simulink model "REFvsFI"  (R2023a)
settings: Solver=FixedStepAuto  StartTime=0.0  StopTime=T  RelTol=1e-3  EnableMultiTasking=on
values from neighbouring files (symbols this model uses):
  Ts = 1    [TestDataGen.m]
libraries: My_FI_Operations x114, simulink x2
(part 4 of 5)

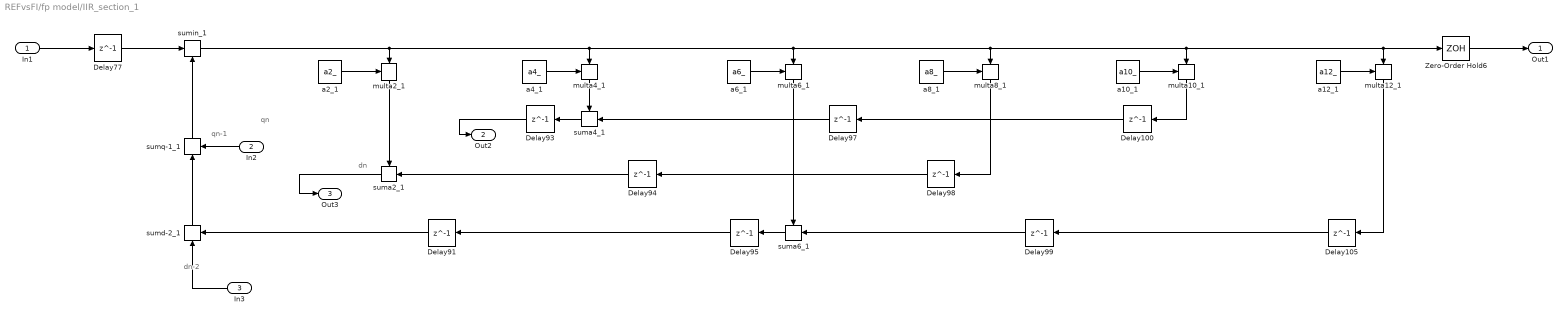
== system REFvsFI/fp model/IIR_section_1 ==
  note: dn
  note: dn-2
  note: qn
  note: qn-1
  In1 : Inport
  In2 : Inport  Port=2
  In3 : Inport  Port=3
  Delay{77,91,93..95,97..100,105} (10 alike) : Delay  DelayLength=1  SampleTime=3*Ts
  Zero-Order Hold6 : ZeroOrderHold  SampleTime=3*Ts
  a10_1 : My_FI_Operations/a10_  SystemSampleTime=-1  VariantActivationTime=update diagram  Latency=0  AutoFrameSizeCalculation=off
  a12_1 : My_FI_Operations/a12_  SystemSampleTime=-1  VariantActivationTime=update diagram  Latency=0  AutoFrameSizeCalculation=off
  a2_1 : My_FI_Operations/a2_  SystemSampleTime=-1  VariantActivationTime=update diagram  Latency=0  AutoFrameSizeCalculation=off
  a4_1 : My_FI_Operations/a4_  SystemSampleTime=-1  VariantActivationTime=update diagram  Latency=0  AutoFrameSizeCalculation=off
  a6_1 : My_FI_Operations/a6_  SystemSampleTime=-1  VariantActivationTime=update diagram  Latency=0  AutoFrameSizeCalculation=off
  a8_1 : My_FI_Operations/a8_  SystemSampleTime=-1  VariantActivationTime=update diagram  Latency=0  AutoFrameSizeCalculation=off
  multa10_1 : My_FI_Operations/multa10_  SystemSampleTime=-1  VariantActivationTime=update diagram  Latency=0  AutoFrameSizeCalculation=off
      settings: PortSchema="{\"entries\":[{\"content\":{\"sides\":[{\"content\":{\"connectorIds\":[\"In1\"]},\"type\":\"ConnectorPlacement.EquallySpacedRectSide\",\"uuid\":\"423828e0-6700-4575-ac06-a5fb7cb5569f\"},{\"content\":{\"connectorIds\":[],\"side\":\"RIGHT\"},\"type\":\"ConnectorPlacement.EquallySpacedRectSide\",\"uuid\":\"a42db842-eb55-44f2-8f04-0144bc45d908\"},{\"content\":{\"connectorIds\":[\"In2\"],\"side\":\"TOP\"},\"type\":\"ConnectorPlacement.EquallySpacedRectSide\",\"uuid\":\"eef5137d-31f0-46b4-a53b-5aa31464a7f9\"},{\"content\":{\"connectorIds\":[\"Out1\"],\"side\":\"BOTTOM\"},\"type\":\"ConnectorPlacement.EquallySpacedRectSide\",\"uuid\":\"0c804fa9-8d94-49f3-91d8-5fb511150c33\"}]},\"type\":\"ConnectorPlacement.EquallySpacedConnector\",\"uuid\":\"7dd7fe03-b221-4701-a7b2-6552f08320da\"}],\"packageUris\":[\"http://schema.mathworks.com/mf0/Connector/R2020b\"],\"version\":\"1.0\"}"
  multa12_1 : My_FI_Operations/multa12_  SystemSampleTime=-1  VariantActivationTime=update diagram  Latency=0  AutoFrameSizeCalculation=off
      settings: PortSchema="{\"entries\":[{\"content\":{\"sides\":[{\"content\":{\"connectorIds\":[\"In1\"]},\"type\":\"ConnectorPlacement.EquallySpacedRectSide\",\"uuid\":\"423828e0-6700-4575-ac06-a5fb7cb5569f\"},{\"content\":{\"connectorIds\":[],\"side\":\"RIGHT\"},\"type\":\"ConnectorPlacement.EquallySpacedRectSide\",\"uuid\":\"a42db842-eb55-44f2-8f04-0144bc45d908\"},{\"content\":{\"connectorIds\":[\"In2\"],\"side\":\"TOP\"},\"type\":\"ConnectorPlacement.EquallySpacedRectSide\",\"uuid\":\"eef5137d-31f0-46b4-a53b-5aa31464a7f9\"},{\"content\":{\"connectorIds\":[\"Out1\"],\"side\":\"BOTTOM\"},\"type\":\"ConnectorPlacement.EquallySpacedRectSide\",\"uuid\":\"8449918d-02c6-4967-8b4f-9e277713318d\"}]},\"type\":\"ConnectorPlacement.EquallySpacedConnector\",\"uuid\":\"7dd7fe03-b221-4701-a7b2-6552f08320da\"}],\"packageUris\":[\"http://schema.mathworks.com/mf0/Connector/R2020b\"],\"version\":\"1.0\"}"
  multa2_1 : My_FI_Operations/multa2_  SystemSampleTime=-1  VariantActivationTime=update diagram  Latency=0  AutoFrameSizeCalculation=off
      settings: PortSchema="{\"entries\":[{\"content\":{\"sides\":[{\"content\":{\"connectorIds\":[\"In1\"]},\"type\":\"ConnectorPlacement.EquallySpacedRectSide\",\"uuid\":\"423828e0-6700-4575-ac06-a5fb7cb5569f\"},{\"content\":{\"connectorIds\":[],\"side\":\"RIGHT\"},\"type\":\"ConnectorPlacement.EquallySpacedRectSide\",\"uuid\":\"a42db842-eb55-44f2-8f04-0144bc45d908\"},{\"content\":{\"connectorIds\":[\"In2\"],\"side\":\"TOP\"},\"type\":\"ConnectorPlacement.EquallySpacedRectSide\",\"uuid\":\"eef5137d-31f0-46b4-a53b-5aa31464a7f9\"},{\"content\":{\"connectorIds\":[\"Out1\"],\"side\":\"BOTTOM\"},\"type\":\"ConnectorPlacement.EquallySpacedRectSide\",\"uuid\":\"55d96b2a-2b7e-4fdf-a401-8e78f7d2a1aa\"}]},\"type\":\"ConnectorPlacement.EquallySpacedConnector\",\"uuid\":\"7dd7fe03-b221-4701-a7b2-6552f08320da\"}],\"packageUris\":[\"http://schema.mathworks.com/mf0/Connector/R2020b\"],\"version\":\"1.0\"}"
  multa4_1 : My_FI_Operations/multa4_  SystemSampleTime=-1  VariantActivationTime=update diagram  Latency=0  AutoFrameSizeCalculation=off
      settings: PortSchema="{\"entries\":[{\"content\":{\"sides\":[{\"content\":{\"connectorIds\":[\"In1\"]},\"type\":\"ConnectorPlacement.EquallySpacedRectSide\",\"uuid\":\"423828e0-6700-4575-ac06-a5fb7cb5569f\"},{\"content\":{\"connectorIds\":[],\"side\":\"RIGHT\"},\"type\":\"ConnectorPlacement.EquallySpacedRectSide\",\"uuid\":\"a42db842-eb55-44f2-8f04-0144bc45d908\"},{\"content\":{\"connectorIds\":[\"In2\"],\"side\":\"TOP\"},\"type\":\"ConnectorPlacement.EquallySpacedRectSide\",\"uuid\":\"eef5137d-31f0-46b4-a53b-5aa31464a7f9\"},{\"content\":{\"connectorIds\":[\"Out1\"],\"side\":\"BOTTOM\"},\"type\":\"ConnectorPlacement.EquallySpacedRectSide\",\"uuid\":\"24a9476e-4370-431a-bbc5-245c90c7a6e7\"}]},\"type\":\"ConnectorPlacement.EquallySpacedConnector\",\"uuid\":\"7dd7fe03-b221-4701-a7b2-6552f08320da\"}],\"packageUris\":[\"http://schema.mathworks.com/mf0/Connector/R2020b\"],\"version\":\"1.0\"}"
  multa6_1 : My_FI_Operations/multa6_  SystemSampleTime=-1  VariantActivationTime=update diagram  Latency=0  AutoFrameSizeCalculation=off
      settings: PortSchema="{\"entries\":[{\"content\":{\"sides\":[{\"content\":{\"connectorIds\":[\"In1\"]},\"type\":\"ConnectorPlacement.EquallySpacedRectSide\",\"uuid\":\"423828e0-6700-4575-ac06-a5fb7cb5569f\"},{\"content\":{\"connectorIds\":[],\"side\":\"RIGHT\"},\"type\":\"ConnectorPlacement.EquallySpacedRectSide\",\"uuid\":\"a42db842-eb55-44f2-8f04-0144bc45d908\"},{\"content\":{\"connectorIds\":[\"In2\"],\"side\":\"TOP\"},\"type\":\"ConnectorPlacement.EquallySpacedRectSide\",\"uuid\":\"eef5137d-31f0-46b4-a53b-5aa31464a7f9\"},{\"content\":{\"connectorIds\":[\"Out1\"],\"side\":\"BOTTOM\"},\"type\":\"ConnectorPlacement.EquallySpacedRectSide\",\"uuid\":\"47329aef-84bb-47a0-9b32-b12909a392a1\"}]},\"type\":\"ConnectorPlacement.EquallySpacedConnector\",\"uuid\":\"7dd7fe03-b221-4701-a7b2-6552f08320da\"}],\"packageUris\":[\"http://schema.mathworks.com/mf0/Connector/R2020b\"],\"version\":\"1.0\"}"
  multa8_1 : My_FI_Operations/multa8_  SystemSampleTime=-1  VariantActivationTime=update diagram  Latency=0  AutoFrameSizeCalculation=off
      settings: PortSchema="{\"entries\":[{\"content\":{\"sides\":[{\"content\":{\"connectorIds\":[\"In1\"]},\"type\":\"ConnectorPlacement.EquallySpacedRectSide\",\"uuid\":\"423828e0-6700-4575-ac06-a5fb7cb5569f\"},{\"content\":{\"connectorIds\":[],\"side\":\"RIGHT\"},\"type\":\"ConnectorPlacement.EquallySpacedRectSide\",\"uuid\":\"a42db842-eb55-44f2-8f04-0144bc45d908\"},{\"content\":{\"connectorIds\":[\"In2\"],\"side\":\"TOP\"},\"type\":\"ConnectorPlacement.EquallySpacedRectSide\",\"uuid\":\"eef5137d-31f0-46b4-a53b-5aa31464a7f9\"},{\"content\":{\"connectorIds\":[\"Out1\"],\"side\":\"BOTTOM\"},\"type\":\"ConnectorPlacement.EquallySpacedRectSide\",\"uuid\":\"5c073f60-f22f-4cd7-abc5-d0d5f88f0213\"}]},\"type\":\"ConnectorPlacement.EquallySpacedConnector\",\"uuid\":\"7dd7fe03-b221-4701-a7b2-6552f08320da\"}],\"packageUris\":[\"http://schema.mathworks.com/mf0/Connector/R2020b\"],\"version\":\"1.0\"}"
  suma2_1 : My_FI_Operations/suma2_  SystemSampleTime=-1  VariantActivationTime=update diagram  Latency=0  AutoFrameSizeCalculation=off
      settings: PortSchema="{\"entries\":[{\"content\":{\"sides\":[{\"content\":{\"connectorIds\":[\"Out1\"]},\"type\":\"ConnectorPlacement.EquallySpacedRectSide\",\"uuid\":\"423828e0-6700-4575-ac06-a5fb7cb5569f\"},{\"content\":{\"connectorIds\":[\"In2\"],\"side\":\"RIGHT\"},\"type\":\"ConnectorPlacement.EquallySpacedRectSide\",\"uuid\":\"a42db842-eb55-44f2-8f04-0144bc45d908\"},{\"content\":{\"connectorIds\":[\"In1\"],\"side\":\"TOP\"},\"type\":\"ConnectorPlacement.EquallySpacedRectSide\",\"uuid\":\"eef5137d-31f0-46b4-a53b-5aa31464a7f9\"}]},\"type\":\"ConnectorPlacement.EquallySpacedConnector\",\"uuid\":\"7dd7fe03-b221-4701-a7b2-6552f08320da\"}],\"packageUris\":[\"http://schema.mathworks.com/mf0/Connector/R2020b\"],\"version\":\"1.0\"}"
  suma4_1 : My_FI_Operations/suma4_  SystemSampleTime=-1  VariantActivationTime=update diagram  Latency=0  AutoFrameSizeCalculation=off
      settings: PortSchema="{\"entries\":[{\"content\":{\"sides\":[{\"content\":{\"connectorIds\":[\"Out1\"]},\"type\":\"ConnectorPlacement.EquallySpacedRectSide\",\"uuid\":\"423828e0-6700-4575-ac06-a5fb7cb5569f\"},{\"content\":{\"connectorIds\":[\"In2\"],\"side\":\"RIGHT\"},\"type\":\"ConnectorPlacement.EquallySpacedRectSide\",\"uuid\":\"a42db842-eb55-44f2-8f04-0144bc45d908\"},{\"content\":{\"connectorIds\":[\"In1\"],\"side\":\"TOP\"},\"type\":\"ConnectorPlacement.EquallySpacedRectSide\",\"uuid\":\"eef5137d-31f0-46b4-a53b-5aa31464a7f9\"}]},\"type\":\"ConnectorPlacement.EquallySpacedConnector\",\"uuid\":\"7dd7fe03-b221-4701-a7b2-6552f08320da\"}],\"packageUris\":[\"http://schema.mathworks.com/mf0/Connector/R2020b\"],\"version\":\"1.0\"}"
  suma6_1 : My_FI_Operations/suma6_  SystemSampleTime=-1  VariantActivationTime=update diagram  Latency=0  AutoFrameSizeCalculation=off
      settings: PortSchema="{\"entries\":[{\"content\":{\"sides\":[{\"content\":{\"connectorIds\":[\"Out1\"]},\"type\":\"ConnectorPlacement.EquallySpacedRectSide\",\"uuid\":\"423828e0-6700-4575-ac06-a5fb7cb5569f\"},{\"content\":{\"connectorIds\":[\"In2\"],\"side\":\"RIGHT\"},\"type\":\"ConnectorPlacement.EquallySpacedRectSide\",\"uuid\":\"a42db842-eb55-44f2-8f04-0144bc45d908\"},{\"content\":{\"connectorIds\":[\"In1\"],\"side\":\"TOP\"},\"type\":\"ConnectorPlacement.EquallySpacedRectSide\",\"uuid\":\"eef5137d-31f0-46b4-a53b-5aa31464a7f9\"}]},\"type\":\"ConnectorPlacement.EquallySpacedConnector\",\"uuid\":\"7dd7fe03-b221-4701-a7b2-6552f08320da\"}],\"packageUris\":[\"http://schema.mathworks.com/mf0/Connector/R2020b\"],\"version\":\"1.0\"}"
  sumd-2_1 : My_FI_Operations/sumd-2_  SystemSampleTime=-1  VariantActivationTime=update diagram  Latency=0  AutoFrameSizeCalculation=off
      settings: PortSchema="{\"entries\":[{\"content\":{\"sides\":[{\"content\":{\"connectorIds\":[]},\"type\":\"ConnectorPlacement.EquallySpacedRectSide\",\"uuid\":\"423828e0-6700-4575-ac06-a5fb7cb5569f\"},{\"content\":{\"connectorIds\":[\"In2\"],\"side\":\"RIGHT\"},\"type\":\"ConnectorPlacement.EquallySpacedRectSide\",\"uuid\":\"a42db842-eb55-44f2-8f04-0144bc45d908\"},{\"content\":{\"connectorIds\":[\"Out1\"],\"side\":\"TOP\"},\"type\":\"ConnectorPlacement.EquallySpacedRectSide\",\"uuid\":\"eef5137d-31f0-46b4-a53b-5aa31464a7f9\"},{\"content\":{\"connectorIds\":[\"In1\"],\"side\":\"BOTTOM\"},\"type\":\"ConnectorPlacement.EquallySpacedRectSide\",\"uuid\":\"0a29e77a-4bdf-45d0-8a25-1103c3446174\"}]},\"type\":\"ConnectorPlacement.EquallySpacedConnector\",\"uuid\":\"7dd7fe03-b221-4701-a7b2-6552f08320da\"}],\"packageUris\":[\"http://schema.mathworks.com/mf0/Connector/R2020b\"],\"version\":\"1.0\"}"
  sumin_1 : My_FI_Operations/sumin_  SystemSampleTime=-1  VariantActivationTime=update diagram  Latency=0  AutoFrameSizeCalculation=off
      settings: PortSchema="{\"entries\":[{\"content\":{\"sides\":[{\"content\":{\"connectorIds\":[\"In1\"]},\"type\":\"ConnectorPlacement.EquallySpacedRectSide\",\"uuid\":\"423828e0-6700-4575-ac06-a5fb7cb5569f\"},{\"content\":{\"connectorIds\":[\"Out1\"],\"side\":\"RIGHT\"},\"type\":\"ConnectorPlacement.EquallySpacedRectSide\",\"uuid\":\"a42db842-eb55-44f2-8f04-0144bc45d908\"},{\"content\":{\"connectorIds\":[],\"side\":\"TOP\"},\"type\":\"ConnectorPlacement.EquallySpacedRectSide\",\"uuid\":\"eef5137d-31f0-46b4-a53b-5aa31464a7f9\"},{\"content\":{\"connectorIds\":[\"In2\"],\"side\":\"BOTTOM\"},\"type\":\"ConnectorPlacement.EquallySpacedRectSide\",\"uuid\":\"f3760898-0e2b-4385-8757-2cc61988fa54\"}]},\"type\":\"ConnectorPlacement.EquallySpacedConnector\",\"uuid\":\"7dd7fe03-b221-4701-a7b2-6552f08320da\"}],\"packageUris\":[\"http://schema.mathworks.com/mf0/Connector/R2020b\"],\"version\":\"1.0\"}"
  sumq-1_1 : My_FI_Operations/sumq-1_  SystemSampleTime=-1  VariantActivationTime=update diagram  Latency=0  AutoFrameSizeCalculation=off
      settings: PortSchema="{\"entries\":[{\"content\":{\"sides\":[{\"content\":{\"connectorIds\":[]},\"type\":\"ConnectorPlacement.EquallySpacedRectSide\",\"uuid\":\"423828e0-6700-4575-ac06-a5fb7cb5569f\"},{\"content\":{\"connectorIds\":[\"In2\"],\"side\":\"RIGHT\"},\"type\":\"ConnectorPlacement.EquallySpacedRectSide\",\"uuid\":\"a42db842-eb55-44f2-8f04-0144bc45d908\"},{\"content\":{\"connectorIds\":[\"Out1\"],\"side\":\"TOP\"},\"type\":\"ConnectorPlacement.EquallySpacedRectSide\",\"uuid\":\"eef5137d-31f0-46b4-a53b-5aa31464a7f9\"},{\"content\":{\"connectorIds\":[\"In1\"],\"side\":\"BOTTOM\"},\"type\":\"ConnectorPlacement.EquallySpacedRectSide\",\"uuid\":\"2873f229-5340-47da-9b40-109923f96826\"}]},\"type\":\"ConnectorPlacement.EquallySpacedConnector\",\"uuid\":\"7dd7fe03-b221-4701-a7b2-6552f08320da\"}],\"packageUris\":[\"http://schema.mathworks.com/mf0/Connector/R2020b\"],\"version\":\"1.0\"}"
  Out1 : Outport
  Out2 : Outport  Port=2
  Out3 : Outport  Port=3
  wires:
  Delay77/1 -> sumin_1/1
  a12_1/1 -> multa12_1/1
  Delay98/1 -> Delay94/1
  Delay91/1 -> sumd-2_1/2
  sumin_1/1 -> multa2_1/2, multa4_1/2, multa6_1/2, multa8_1/2, multa10_1/2, multa12_1/2, Zero-Order Hold6/1
  Delay99/1 -> suma6_1/2
  Delay95/1 -> Delay91/1
  Delay94/1 -> suma2_1/2
  sumd-2_1/1 -> sumq-1_1/1
  a2_1/1 -> multa2_1/1
  multa4_1/1 -> suma4_1/1
  Delay100/1 -> Delay97/1
  Zero-Order Hold6/1 -> Out1/1
  multa6_1/1 -> suma6_1/1
  a10_1/1 -> multa10_1/1
  a4_1/1 -> multa4_1/1
  multa12_1/1 -> Delay105/1
  multa2_1/1 -> suma2_1/1
  Delay105/1 -> Delay99/1
  a8_1/1 -> multa8_1/1
  suma6_1/1 -> Delay95/1
  Delay97/1 -> suma4_1/2
  multa10_1/1 -> Delay100/1
  suma4_1/1 -> Delay93/1
  multa8_1/1 -> Delay98/1
  Delay93/1 -> Out2/1
  sumq-1_1/1 -> sumin_1/2
  a6_1/1 -> multa6_1/1
  In2/1 -> sumq-1_1/2
  In1/1 -> Delay77/1
  In3/1 -> sumd-2_1/1
  suma2_1/1 -> Out3/1

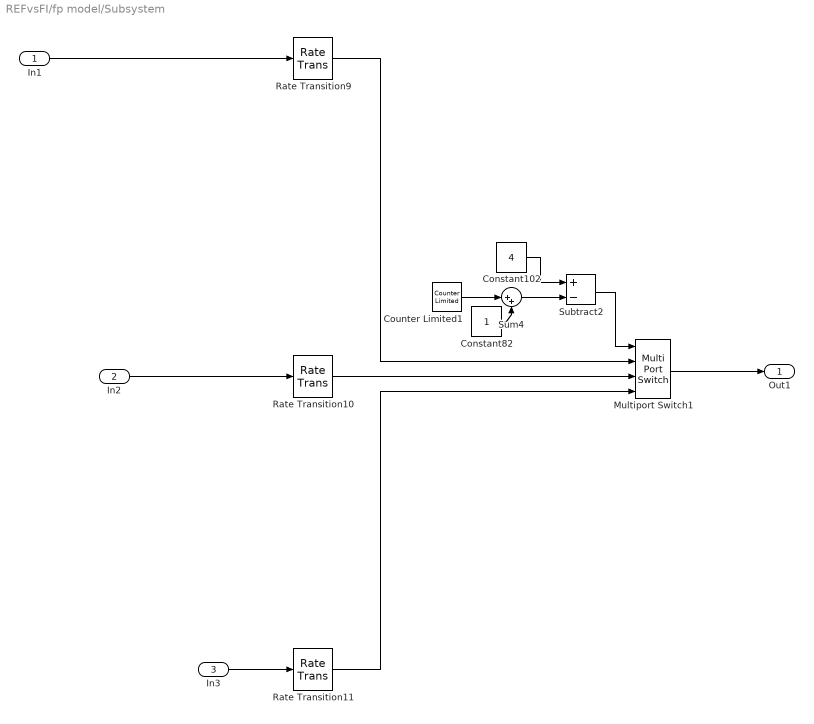
== system REFvsFI/fp model/Subsystem ==
  In1 : Inport
  In2 : Inport  Port=2
  In3 : Inport  Port=3
  Constant102 : Constant  Value=4  OutDataTypeStr=fixdt(0,3,0)
  Constant82 : Constant  OutDataTypeStr=fixdt(0,1,0)
  Counter Limited1 : simulink/Sources/Counter Limited  uplimit=2  tsamp=Ts
  Multiport Switch1 : MultiPortSwitch  OutDataTypeStr=fixdt(1,WL,FLout)  RndMeth=Nearest  SaturateOnIntegerOverflow=off  InputSameDT=off
  Rate Transition10 : RateTransition  OutPortSampleTime=Ts
  Rate Transition11 : RateTransition  OutPortSampleTime=Ts
  Rate Transition9 : RateTransition  OutPortSampleTime=Ts
  Subtract2 : Sum  Inputs=+-  OutDataTypeStr=fixdt(0,2,0)
  Sum4 : Sum  Inputs=|++  OutDataTypeStr=fixdt(0,2,0)
  Out1 : Outport
  wires:
  Rate Transition11/1 -> Multiport Switch1/4
  Constant82/1 -> Sum4/2
  Subtract2/1 -> Multiport Switch1/1
  Counter Limited1/1 -> Sum4/1
  Sum4/1 -> Subtract2/2
  Constant102/1 -> Subtract2/1
  Rate Transition9/1 -> Multiport Switch1/2
  Rate Transition10/1 -> Multiport Switch1/3
  In2/1 -> Rate Transition10/1
  In1/1 -> Rate Transition9/1
  Multiport Switch1/1 -> Out1/1
  In3/1 -> Rate Transition11/1

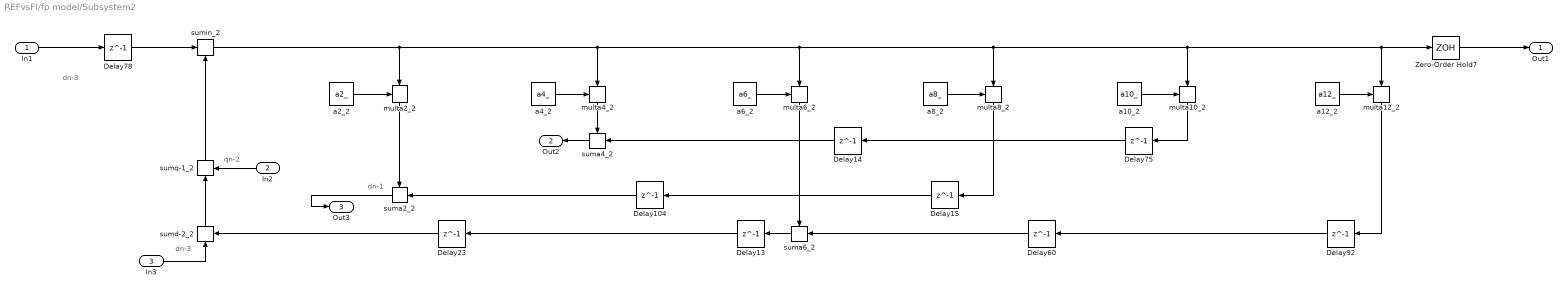
== system REFvsFI/fp model/Subsystem2 ==
  note: dn-1
  note: dn-3
  note: dn-3
  note: qn-2
  In1 : Inport
  In2 : Inport  Port=2
  In3 : Inport  Port=3
  Delay{13..15,23,60,75,78,92,104} (9 alike) : Delay  DelayLength=1  SampleTime=3*Ts
  Zero-Order Hold7 : ZeroOrderHold  SampleTime=3*Ts
  a10_2 : My_FI_Operations/a10_  SystemSampleTime=-1  VariantActivationTime=update diagram  Latency=0  AutoFrameSizeCalculation=off
  a12_2 : My_FI_Operations/a12_  SystemSampleTime=-1  VariantActivationTime=update diagram  Latency=0  AutoFrameSizeCalculation=off
  a2_2 : My_FI_Operations/a2_  SystemSampleTime=-1  VariantActivationTime=update diagram  Latency=0  AutoFrameSizeCalculation=off
  a4_2 : My_FI_Operations/a4_  SystemSampleTime=-1  VariantActivationTime=update diagram  Latency=0  AutoFrameSizeCalculation=off
  a6_2 : My_FI_Operations/a6_  SystemSampleTime=-1  VariantActivationTime=update diagram  Latency=0  AutoFrameSizeCalculation=off
  a8_2 : My_FI_Operations/a8_  SystemSampleTime=-1  VariantActivationTime=update diagram  Latency=0  AutoFrameSizeCalculation=off
  multa10_2 : My_FI_Operations/multa10_  SystemSampleTime=-1  VariantActivationTime=update diagram  Latency=0  AutoFrameSizeCalculation=off
      settings: PortSchema="{\"entries\":[{\"content\":{\"sides\":[{\"content\":{\"connectorIds\":[\"In1\"]},\"type\":\"ConnectorPlacement.EquallySpacedRectSide\",\"uuid\":\"423828e0-6700-4575-ac06-a5fb7cb5569f\"},{\"content\":{\"connectorIds\":[],\"side\":\"RIGHT\"},\"type\":\"ConnectorPlacement.EquallySpacedRectSide\",\"uuid\":\"a42db842-eb55-44f2-8f04-0144bc45d908\"},{\"content\":{\"connectorIds\":[\"In2\"],\"side\":\"TOP\"},\"type\":\"ConnectorPlacement.EquallySpacedRectSide\",\"uuid\":\"eef5137d-31f0-46b4-a53b-5aa31464a7f9\"},{\"content\":{\"connectorIds\":[\"Out1\"],\"side\":\"BOTTOM\"},\"type\":\"ConnectorPlacement.EquallySpacedRectSide\",\"uuid\":\"0c804fa9-8d94-49f3-91d8-5fb511150c33\"}]},\"type\":\"ConnectorPlacement.EquallySpacedConnector\",\"uuid\":\"7dd7fe03-b221-4701-a7b2-6552f08320da\"}],\"packageUris\":[\"http://schema.mathworks.com/mf0/Connector/R2020b\"],\"version\":\"1.0\"}"
  multa12_2 : My_FI_Operations/multa12_  SystemSampleTime=-1  VariantActivationTime=update diagram  Latency=0  AutoFrameSizeCalculation=off
      settings: PortSchema="{\"entries\":[{\"content\":{\"sides\":[{\"content\":{\"connectorIds\":[\"In1\"]},\"type\":\"ConnectorPlacement.EquallySpacedRectSide\",\"uuid\":\"423828e0-6700-4575-ac06-a5fb7cb5569f\"},{\"content\":{\"connectorIds\":[],\"side\":\"RIGHT\"},\"type\":\"ConnectorPlacement.EquallySpacedRectSide\",\"uuid\":\"a42db842-eb55-44f2-8f04-0144bc45d908\"},{\"content\":{\"connectorIds\":[\"In2\"],\"side\":\"TOP\"},\"type\":\"ConnectorPlacement.EquallySpacedRectSide\",\"uuid\":\"eef5137d-31f0-46b4-a53b-5aa31464a7f9\"},{\"content\":{\"connectorIds\":[\"Out1\"],\"side\":\"BOTTOM\"},\"type\":\"ConnectorPlacement.EquallySpacedRectSide\",\"uuid\":\"8449918d-02c6-4967-8b4f-9e277713318d\"}]},\"type\":\"ConnectorPlacement.EquallySpacedConnector\",\"uuid\":\"7dd7fe03-b221-4701-a7b2-6552f08320da\"}],\"packageUris\":[\"http://schema.mathworks.com/mf0/Connector/R2020b\"],\"version\":\"1.0\"}"
  multa2_2 : My_FI_Operations/multa2_  SystemSampleTime=-1  VariantActivationTime=update diagram  Latency=0  AutoFrameSizeCalculation=off
      settings: PortSchema="{\"entries\":[{\"content\":{\"sides\":[{\"content\":{\"connectorIds\":[\"In1\"]},\"type\":\"ConnectorPlacement.EquallySpacedRectSide\",\"uuid\":\"423828e0-6700-4575-ac06-a5fb7cb5569f\"},{\"content\":{\"connectorIds\":[],\"side\":\"RIGHT\"},\"type\":\"ConnectorPlacement.EquallySpacedRectSide\",\"uuid\":\"a42db842-eb55-44f2-8f04-0144bc45d908\"},{\"content\":{\"connectorIds\":[\"In2\"],\"side\":\"TOP\"},\"type\":\"ConnectorPlacement.EquallySpacedRectSide\",\"uuid\":\"eef5137d-31f0-46b4-a53b-5aa31464a7f9\"},{\"content\":{\"connectorIds\":[\"Out1\"],\"side\":\"BOTTOM\"},\"type\":\"ConnectorPlacement.EquallySpacedRectSide\",\"uuid\":\"55d96b2a-2b7e-4fdf-a401-8e78f7d2a1aa\"}]},\"type\":\"ConnectorPlacement.EquallySpacedConnector\",\"uuid\":\"7dd7fe03-b221-4701-a7b2-6552f08320da\"}],\"packageUris\":[\"http://schema.mathworks.com/mf0/Connector/R2020b\"],\"version\":\"1.0\"}"
  multa4_2 : My_FI_Operations/multa4_  SystemSampleTime=-1  VariantActivationTime=update diagram  Latency=0  AutoFrameSizeCalculation=off
      settings: PortSchema="{\"entries\":[{\"content\":{\"sides\":[{\"content\":{\"connectorIds\":[\"In1\"]},\"type\":\"ConnectorPlacement.EquallySpacedRectSide\",\"uuid\":\"423828e0-6700-4575-ac06-a5fb7cb5569f\"},{\"content\":{\"connectorIds\":[],\"side\":\"RIGHT\"},\"type\":\"ConnectorPlacement.EquallySpacedRectSide\",\"uuid\":\"a42db842-eb55-44f2-8f04-0144bc45d908\"},{\"content\":{\"connectorIds\":[\"In2\"],\"side\":\"TOP\"},\"type\":\"ConnectorPlacement.EquallySpacedRectSide\",\"uuid\":\"eef5137d-31f0-46b4-a53b-5aa31464a7f9\"},{\"content\":{\"connectorIds\":[\"Out1\"],\"side\":\"BOTTOM\"},\"type\":\"ConnectorPlacement.EquallySpacedRectSide\",\"uuid\":\"24a9476e-4370-431a-bbc5-245c90c7a6e7\"}]},\"type\":\"ConnectorPlacement.EquallySpacedConnector\",\"uuid\":\"7dd7fe03-b221-4701-a7b2-6552f08320da\"}],\"packageUris\":[\"http://schema.mathworks.com/mf0/Connector/R2020b\"],\"version\":\"1.0\"}"
  multa6_2 : My_FI_Operations/multa6_  SystemSampleTime=-1  VariantActivationTime=update diagram  Latency=0  AutoFrameSizeCalculation=off
      settings: PortSchema="{\"entries\":[{\"content\":{\"sides\":[{\"content\":{\"connectorIds\":[\"In1\"]},\"type\":\"ConnectorPlacement.EquallySpacedRectSide\",\"uuid\":\"423828e0-6700-4575-ac06-a5fb7cb5569f\"},{\"content\":{\"connectorIds\":[],\"side\":\"RIGHT\"},\"type\":\"ConnectorPlacement.EquallySpacedRectSide\",\"uuid\":\"a42db842-eb55-44f2-8f04-0144bc45d908\"},{\"content\":{\"connectorIds\":[\"In2\"],\"side\":\"TOP\"},\"type\":\"ConnectorPlacement.EquallySpacedRectSide\",\"uuid\":\"eef5137d-31f0-46b4-a53b-5aa31464a7f9\"},{\"content\":{\"connectorIds\":[\"Out1\"],\"side\":\"BOTTOM\"},\"type\":\"ConnectorPlacement.EquallySpacedRectSide\",\"uuid\":\"47329aef-84bb-47a0-9b32-b12909a392a1\"}]},\"type\":\"ConnectorPlacement.EquallySpacedConnector\",\"uuid\":\"7dd7fe03-b221-4701-a7b2-6552f08320da\"}],\"packageUris\":[\"http://schema.mathworks.com/mf0/Connector/R2020b\"],\"version\":\"1.0\"}"
  multa8_2 : My_FI_Operations/multa8_  SystemSampleTime=-1  VariantActivationTime=update diagram  Latency=0  AutoFrameSizeCalculation=off
      settings: PortSchema="{\"entries\":[{\"content\":{\"sides\":[{\"content\":{\"connectorIds\":[\"In1\"]},\"type\":\"ConnectorPlacement.EquallySpacedRectSide\",\"uuid\":\"423828e0-6700-4575-ac06-a5fb7cb5569f\"},{\"content\":{\"connectorIds\":[],\"side\":\"RIGHT\"},\"type\":\"ConnectorPlacement.EquallySpacedRectSide\",\"uuid\":\"a42db842-eb55-44f2-8f04-0144bc45d908\"},{\"content\":{\"connectorIds\":[\"In2\"],\"side\":\"TOP\"},\"type\":\"ConnectorPlacement.EquallySpacedRectSide\",\"uuid\":\"eef5137d-31f0-46b4-a53b-5aa31464a7f9\"},{\"content\":{\"connectorIds\":[\"Out1\"],\"side\":\"BOTTOM\"},\"type\":\"ConnectorPlacement.EquallySpacedRectSide\",\"uuid\":\"5c073f60-f22f-4cd7-abc5-d0d5f88f0213\"}]},\"type\":\"ConnectorPlacement.EquallySpacedConnector\",\"uuid\":\"7dd7fe03-b221-4701-a7b2-6552f08320da\"}],\"packageUris\":[\"http://schema.mathworks.com/mf0/Connector/R2020b\"],\"version\":\"1.0\"}"
  suma2_2 : My_FI_Operations/suma2_  SystemSampleTime=-1  VariantActivationTime=update diagram  Latency=0  AutoFrameSizeCalculation=off
      settings: PortSchema="{\"entries\":[{\"content\":{\"sides\":[{\"content\":{\"connectorIds\":[\"Out1\"]},\"type\":\"ConnectorPlacement.EquallySpacedRectSide\",\"uuid\":\"423828e0-6700-4575-ac06-a5fb7cb5569f\"},{\"content\":{\"connectorIds\":[\"In2\"],\"side\":\"RIGHT\"},\"type\":\"ConnectorPlacement.EquallySpacedRectSide\",\"uuid\":\"a42db842-eb55-44f2-8f04-0144bc45d908\"},{\"content\":{\"connectorIds\":[\"In1\"],\"side\":\"TOP\"},\"type\":\"ConnectorPlacement.EquallySpacedRectSide\",\"uuid\":\"eef5137d-31f0-46b4-a53b-5aa31464a7f9\"}]},\"type\":\"ConnectorPlacement.EquallySpacedConnector\",\"uuid\":\"7dd7fe03-b221-4701-a7b2-6552f08320da\"}],\"packageUris\":[\"http://schema.mathworks.com/mf0/Connector/R2020b\"],\"version\":\"1.0\"}"
  suma4_2 : My_FI_Operations/suma4_  SystemSampleTime=-1  VariantActivationTime=update diagram  Latency=0  AutoFrameSizeCalculation=off
      settings: PortSchema="{\"entries\":[{\"content\":{\"sides\":[{\"content\":{\"connectorIds\":[\"Out1\"]},\"type\":\"ConnectorPlacement.EquallySpacedRectSide\",\"uuid\":\"423828e0-6700-4575-ac06-a5fb7cb5569f\"},{\"content\":{\"connectorIds\":[\"In2\"],\"side\":\"RIGHT\"},\"type\":\"ConnectorPlacement.EquallySpacedRectSide\",\"uuid\":\"a42db842-eb55-44f2-8f04-0144bc45d908\"},{\"content\":{\"connectorIds\":[\"In1\"],\"side\":\"TOP\"},\"type\":\"ConnectorPlacement.EquallySpacedRectSide\",\"uuid\":\"eef5137d-31f0-46b4-a53b-5aa31464a7f9\"}]},\"type\":\"ConnectorPlacement.EquallySpacedConnector\",\"uuid\":\"7dd7fe03-b221-4701-a7b2-6552f08320da\"}],\"packageUris\":[\"http://schema.mathworks.com/mf0/Connector/R2020b\"],\"version\":\"1.0\"}"
  suma6_2 : My_FI_Operations/suma6_  SystemSampleTime=-1  VariantActivationTime=update diagram  Latency=0  AutoFrameSizeCalculation=off
      settings: PortSchema="{\"entries\":[{\"content\":{\"sides\":[{\"content\":{\"connectorIds\":[\"Out1\"]},\"type\":\"ConnectorPlacement.EquallySpacedRectSide\",\"uuid\":\"423828e0-6700-4575-ac06-a5fb7cb5569f\"},{\"content\":{\"connectorIds\":[\"In2\"],\"side\":\"RIGHT\"},\"type\":\"ConnectorPlacement.EquallySpacedRectSide\",\"uuid\":\"a42db842-eb55-44f2-8f04-0144bc45d908\"},{\"content\":{\"connectorIds\":[\"In1\"],\"side\":\"TOP\"},\"type\":\"ConnectorPlacement.EquallySpacedRectSide\",\"uuid\":\"eef5137d-31f0-46b4-a53b-5aa31464a7f9\"}]},\"type\":\"ConnectorPlacement.EquallySpacedConnector\",\"uuid\":\"7dd7fe03-b221-4701-a7b2-6552f08320da\"}],\"packageUris\":[\"http://schema.mathworks.com/mf0/Connector/R2020b\"],\"version\":\"1.0\"}"
  sumd-2_2 : My_FI_Operations/sumd-2_  SystemSampleTime=-1  VariantActivationTime=update diagram  Latency=0  AutoFrameSizeCalculation=off
      settings: PortSchema="{\"entries\":[{\"content\":{\"sides\":[{\"content\":{\"connectorIds\":[]},\"type\":\"ConnectorPlacement.EquallySpacedRectSide\",\"uuid\":\"423828e0-6700-4575-ac06-a5fb7cb5569f\"},{\"content\":{\"connectorIds\":[\"In2\"],\"side\":\"RIGHT\"},\"type\":\"ConnectorPlacement.EquallySpacedRectSide\",\"uuid\":\"a42db842-eb55-44f2-8f04-0144bc45d908\"},{\"content\":{\"connectorIds\":[\"Out1\"],\"side\":\"TOP\"},\"type\":\"ConnectorPlacement.EquallySpacedRectSide\",\"uuid\":\"eef5137d-31f0-46b4-a53b-5aa31464a7f9\"},{\"content\":{\"connectorIds\":[\"In1\"],\"side\":\"BOTTOM\"},\"type\":\"ConnectorPlacement.EquallySpacedRectSide\",\"uuid\":\"0a29e77a-4bdf-45d0-8a25-1103c3446174\"}]},\"type\":\"ConnectorPlacement.EquallySpacedConnector\",\"uuid\":\"7dd7fe03-b221-4701-a7b2-6552f08320da\"}],\"packageUris\":[\"http://schema.mathworks.com/mf0/Connector/R2020b\"],\"version\":\"1.0\"}"
  sumin_2 : My_FI_Operations/sumin_  SystemSampleTime=-1  VariantActivationTime=update diagram  Latency=0  AutoFrameSizeCalculation=off
      settings: PortSchema="{\"entries\":[{\"content\":{\"sides\":[{\"content\":{\"connectorIds\":[\"In1\"]},\"type\":\"ConnectorPlacement.EquallySpacedRectSide\",\"uuid\":\"423828e0-6700-4575-ac06-a5fb7cb5569f\"},{\"content\":{\"connectorIds\":[\"Out1\"],\"side\":\"RIGHT\"},\"type\":\"ConnectorPlacement.EquallySpacedRectSide\",\"uuid\":\"a42db842-eb55-44f2-8f04-0144bc45d908\"},{\"content\":{\"connectorIds\":[],\"side\":\"TOP\"},\"type\":\"ConnectorPlacement.EquallySpacedRectSide\",\"uuid\":\"eef5137d-31f0-46b4-a53b-5aa31464a7f9\"},{\"content\":{\"connectorIds\":[\"In2\"],\"side\":\"BOTTOM\"},\"type\":\"ConnectorPlacement.EquallySpacedRectSide\",\"uuid\":\"f3760898-0e2b-4385-8757-2cc61988fa54\"}]},\"type\":\"ConnectorPlacement.EquallySpacedConnector\",\"uuid\":\"7dd7fe03-b221-4701-a7b2-6552f08320da\"}],\"packageUris\":[\"http://schema.mathworks.com/mf0/Connector/R2020b\"],\"version\":\"1.0\"}"
  sumq-1_2 : My_FI_Operations/sumq-1_  SystemSampleTime=-1  VariantActivationTime=update diagram  Latency=0  AutoFrameSizeCalculation=off
      settings: PortSchema="{\"entries\":[{\"content\":{\"sides\":[{\"content\":{\"connectorIds\":[]},\"type\":\"ConnectorPlacement.EquallySpacedRectSide\",\"uuid\":\"423828e0-6700-4575-ac06-a5fb7cb5569f\"},{\"content\":{\"connectorIds\":[\"In2\"],\"side\":\"RIGHT\"},\"type\":\"ConnectorPlacement.EquallySpacedRectSide\",\"uuid\":\"a42db842-eb55-44f2-8f04-0144bc45d908\"},{\"content\":{\"connectorIds\":[\"Out1\"],\"side\":\"TOP\"},\"type\":\"ConnectorPlacement.EquallySpacedRectSide\",\"uuid\":\"eef5137d-31f0-46b4-a53b-5aa31464a7f9\"},{\"content\":{\"connectorIds\":[\"In1\"],\"side\":\"BOTTOM\"},\"type\":\"ConnectorPlacement.EquallySpacedRectSide\",\"uuid\":\"2873f229-5340-47da-9b40-109923f96826\"}]},\"type\":\"ConnectorPlacement.EquallySpacedConnector\",\"uuid\":\"7dd7fe03-b221-4701-a7b2-6552f08320da\"}],\"packageUris\":[\"http://schema.mathworks.com/mf0/Connector/R2020b\"],\"version\":\"1.0\"}"
  Out1 : Outport
  Out2 : Outport  Port=2
  Out3 : Outport  Port=3
  wires:
  sumin_2/1 -> multa2_2/2, multa12_2/2, Zero-Order Hold7/1, multa10_2/2, multa8_2/2, multa6_2/2, multa4_2/2
  In2/1 -> sumq-1_2/2
  a12_2/1 -> multa12_2/1
  Delay78/1 -> sumin_2/1
  sumd-2_2/1 -> sumq-1_2/1
  suma6_2/1 -> Delay13/1
  Zero-Order Hold7/1 -> Out1/1
  sumq-1_2/1 -> sumin_2/2
  Delay15/1 -> Delay104/1
  Delay13/1 -> Delay23/1
  a10_2/1 -> multa10_2/1
  suma4_2/1 -> Out2/1
  In3/1 -> sumd-2_2/1
  multa10_2/1 -> Delay75/1
  multa8_2/1 -> Delay15/1
  multa4_2/1 -> suma4_2/1
  multa2_2/1 -> suma2_2/1
  Delay14/1 -> suma4_2/2
  a2_2/1 -> multa2_2/1
  Delay60/1 -> suma6_2/2
  a8_2/1 -> multa8_2/1
  multa6_2/1 -> suma6_2/1
  Delay75/1 -> Delay14/1
  multa12_2/1 -> Delay92/1
  a4_2/1 -> multa4_2/1
  a6_2/1 -> multa6_2/1
  Delay23/1 -> sumd-2_2/2
  Delay104/1 -> suma2_2/2
  In1/1 -> Delay78/1
  Delay92/1 -> Delay60/1
  suma2_2/1 -> Out3/1

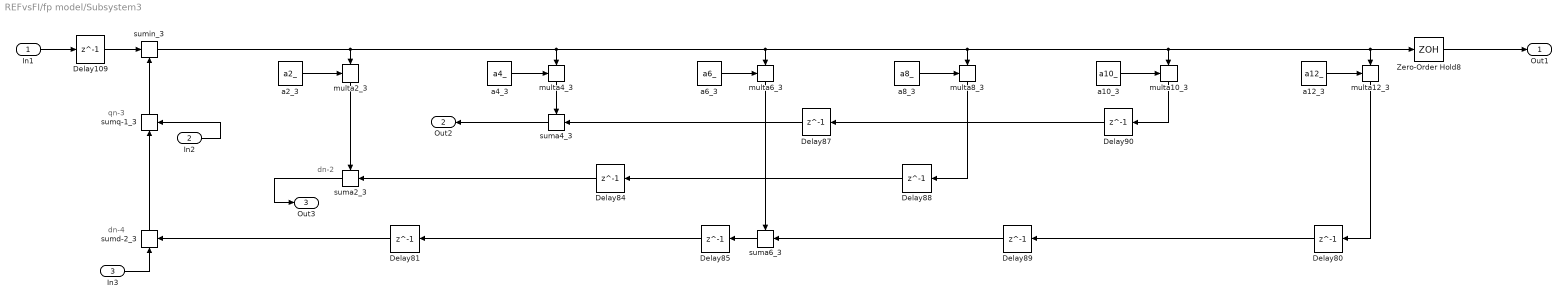
== system REFvsFI/fp model/Subsystem3 ==
  note: dn-2
  note: dn-4
  note: qn-3
  In1 : Inport
  In2 : Inport  Port=2
  In3 : Inport  Port=3
  Delay{80..81,84..85,87..90,109} (9 alike) : Delay  DelayLength=1  SampleTime=3*Ts
  Zero-Order Hold8 : ZeroOrderHold  SampleTime=3*Ts
  a10_3 : My_FI_Operations/a10_  SystemSampleTime=-1  VariantActivationTime=update diagram  Latency=0  AutoFrameSizeCalculation=off
  a12_3 : My_FI_Operations/a12_  SystemSampleTime=-1  VariantActivationTime=update diagram  Latency=0  AutoFrameSizeCalculation=off
  a2_3 : My_FI_Operations/a2_  SystemSampleTime=-1  VariantActivationTime=update diagram  Latency=0  AutoFrameSizeCalculation=off
  a4_3 : My_FI_Operations/a4_  SystemSampleTime=-1  VariantActivationTime=update diagram  Latency=0  AutoFrameSizeCalculation=off
  a6_3 : My_FI_Operations/a6_  SystemSampleTime=-1  VariantActivationTime=update diagram  Latency=0  AutoFrameSizeCalculation=off
  a8_3 : My_FI_Operations/a8_  SystemSampleTime=-1  VariantActivationTime=update diagram  Latency=0  AutoFrameSizeCalculation=off
  multa10_3 : My_FI_Operations/multa10_  SystemSampleTime=-1  VariantActivationTime=update diagram  Latency=0  AutoFrameSizeCalculation=off
      settings: PortSchema="{\"entries\":[{\"content\":{\"sides\":[{\"content\":{\"connectorIds\":[\"In1\"]},\"type\":\"ConnectorPlacement.EquallySpacedRectSide\",\"uuid\":\"423828e0-6700-4575-ac06-a5fb7cb5569f\"},{\"content\":{\"connectorIds\":[],\"side\":\"RIGHT\"},\"type\":\"ConnectorPlacement.EquallySpacedRectSide\",\"uuid\":\"a42db842-eb55-44f2-8f04-0144bc45d908\"},{\"content\":{\"connectorIds\":[\"In2\"],\"side\":\"TOP\"},\"type\":\"ConnectorPlacement.EquallySpacedRectSide\",\"uuid\":\"eef5137d-31f0-46b4-a53b-5aa31464a7f9\"},{\"content\":{\"connectorIds\":[\"Out1\"],\"side\":\"BOTTOM\"},\"type\":\"ConnectorPlacement.EquallySpacedRectSide\",\"uuid\":\"0c804fa9-8d94-49f3-91d8-5fb511150c33\"}]},\"type\":\"ConnectorPlacement.EquallySpacedConnector\",\"uuid\":\"7dd7fe03-b221-4701-a7b2-6552f08320da\"}],\"packageUris\":[\"http://schema.mathworks.com/mf0/Connector/R2020b\"],\"version\":\"1.0\"}"
  multa12_3 : My_FI_Operations/multa12_  SystemSampleTime=-1  VariantActivationTime=update diagram  Latency=0  AutoFrameSizeCalculation=off
      settings: PortSchema="{\"entries\":[{\"content\":{\"sides\":[{\"content\":{\"connectorIds\":[\"In1\"]},\"type\":\"ConnectorPlacement.EquallySpacedRectSide\",\"uuid\":\"423828e0-6700-4575-ac06-a5fb7cb5569f\"},{\"content\":{\"connectorIds\":[],\"side\":\"RIGHT\"},\"type\":\"ConnectorPlacement.EquallySpacedRectSide\",\"uuid\":\"a42db842-eb55-44f2-8f04-0144bc45d908\"},{\"content\":{\"connectorIds\":[\"In2\"],\"side\":\"TOP\"},\"type\":\"ConnectorPlacement.EquallySpacedRectSide\",\"uuid\":\"eef5137d-31f0-46b4-a53b-5aa31464a7f9\"},{\"content\":{\"connectorIds\":[\"Out1\"],\"side\":\"BOTTOM\"},\"type\":\"ConnectorPlacement.EquallySpacedRectSide\",\"uuid\":\"8449918d-02c6-4967-8b4f-9e277713318d\"}]},\"type\":\"ConnectorPlacement.EquallySpacedConnector\",\"uuid\":\"7dd7fe03-b221-4701-a7b2-6552f08320da\"}],\"packageUris\":[\"http://schema.mathworks.com/mf0/Connector/R2020b\"],\"version\":\"1.0\"}"
  multa2_3 : My_FI_Operations/multa2_  SystemSampleTime=-1  VariantActivationTime=update diagram  Latency=0  AutoFrameSizeCalculation=off
      settings: PortSchema="{\"entries\":[{\"content\":{\"sides\":[{\"content\":{\"connectorIds\":[\"In1\"]},\"type\":\"ConnectorPlacement.EquallySpacedRectSide\",\"uuid\":\"423828e0-6700-4575-ac06-a5fb7cb5569f\"},{\"content\":{\"connectorIds\":[],\"side\":\"RIGHT\"},\"type\":\"ConnectorPlacement.EquallySpacedRectSide\",\"uuid\":\"a42db842-eb55-44f2-8f04-0144bc45d908\"},{\"content\":{\"connectorIds\":[\"In2\"],\"side\":\"TOP\"},\"type\":\"ConnectorPlacement.EquallySpacedRectSide\",\"uuid\":\"eef5137d-31f0-46b4-a53b-5aa31464a7f9\"},{\"content\":{\"connectorIds\":[\"Out1\"],\"side\":\"BOTTOM\"},\"type\":\"ConnectorPlacement.EquallySpacedRectSide\",\"uuid\":\"55d96b2a-2b7e-4fdf-a401-8e78f7d2a1aa\"}]},\"type\":\"ConnectorPlacement.EquallySpacedConnector\",\"uuid\":\"7dd7fe03-b221-4701-a7b2-6552f08320da\"}],\"packageUris\":[\"http://schema.mathworks.com/mf0/Connector/R2020b\"],\"version\":\"1.0\"}"
  multa4_3 : My_FI_Operations/multa4_  SystemSampleTime=-1  VariantActivationTime=update diagram  Latency=0  AutoFrameSizeCalculation=off
      settings: PortSchema="{\"entries\":[{\"content\":{\"sides\":[{\"content\":{\"connectorIds\":[\"In1\"]},\"type\":\"ConnectorPlacement.EquallySpacedRectSide\",\"uuid\":\"423828e0-6700-4575-ac06-a5fb7cb5569f\"},{\"content\":{\"connectorIds\":[],\"side\":\"RIGHT\"},\"type\":\"ConnectorPlacement.EquallySpacedRectSide\",\"uuid\":\"a42db842-eb55-44f2-8f04-0144bc45d908\"},{\"content\":{\"connectorIds\":[\"In2\"],\"side\":\"TOP\"},\"type\":\"ConnectorPlacement.EquallySpacedRectSide\",\"uuid\":\"eef5137d-31f0-46b4-a53b-5aa31464a7f9\"},{\"content\":{\"connectorIds\":[\"Out1\"],\"side\":\"BOTTOM\"},\"type\":\"ConnectorPlacement.EquallySpacedRectSide\",\"uuid\":\"24a9476e-4370-431a-bbc5-245c90c7a6e7\"}]},\"type\":\"ConnectorPlacement.EquallySpacedConnector\",\"uuid\":\"7dd7fe03-b221-4701-a7b2-6552f08320da\"}],\"packageUris\":[\"http://schema.mathworks.com/mf0/Connector/R2020b\"],\"version\":\"1.0\"}"
  multa6_3 : My_FI_Operations/multa6_  SystemSampleTime=-1  VariantActivationTime=update diagram  Latency=0  AutoFrameSizeCalculation=off
      settings: PortSchema="{\"entries\":[{\"content\":{\"sides\":[{\"content\":{\"connectorIds\":[\"In1\"]},\"type\":\"ConnectorPlacement.EquallySpacedRectSide\",\"uuid\":\"423828e0-6700-4575-ac06-a5fb7cb5569f\"},{\"content\":{\"connectorIds\":[],\"side\":\"RIGHT\"},\"type\":\"ConnectorPlacement.EquallySpacedRectSide\",\"uuid\":\"a42db842-eb55-44f2-8f04-0144bc45d908\"},{\"content\":{\"connectorIds\":[\"In2\"],\"side\":\"TOP\"},\"type\":\"ConnectorPlacement.EquallySpacedRectSide\",\"uuid\":\"eef5137d-31f0-46b4-a53b-5aa31464a7f9\"},{\"content\":{\"connectorIds\":[\"Out1\"],\"side\":\"BOTTOM\"},\"type\":\"ConnectorPlacement.EquallySpacedRectSide\",\"uuid\":\"47329aef-84bb-47a0-9b32-b12909a392a1\"}]},\"type\":\"ConnectorPlacement.EquallySpacedConnector\",\"uuid\":\"7dd7fe03-b221-4701-a7b2-6552f08320da\"}],\"packageUris\":[\"http://schema.mathworks.com/mf0/Connector/R2020b\"],\"version\":\"1.0\"}"
  multa8_3 : My_FI_Operations/multa8_  SystemSampleTime=-1  VariantActivationTime=update diagram  Latency=0  AutoFrameSizeCalculation=off
      settings: PortSchema="{\"entries\":[{\"content\":{\"sides\":[{\"content\":{\"connectorIds\":[\"In1\"]},\"type\":\"ConnectorPlacement.EquallySpacedRectSide\",\"uuid\":\"423828e0-6700-4575-ac06-a5fb7cb5569f\"},{\"content\":{\"connectorIds\":[],\"side\":\"RIGHT\"},\"type\":\"ConnectorPlacement.EquallySpacedRectSide\",\"uuid\":\"a42db842-eb55-44f2-8f04-0144bc45d908\"},{\"content\":{\"connectorIds\":[\"In2\"],\"side\":\"TOP\"},\"type\":\"ConnectorPlacement.EquallySpacedRectSide\",\"uuid\":\"eef5137d-31f0-46b4-a53b-5aa31464a7f9\"},{\"content\":{\"connectorIds\":[\"Out1\"],\"side\":\"BOTTOM\"},\"type\":\"ConnectorPlacement.EquallySpacedRectSide\",\"uuid\":\"5c073f60-f22f-4cd7-abc5-d0d5f88f0213\"}]},\"type\":\"ConnectorPlacement.EquallySpacedConnector\",\"uuid\":\"7dd7fe03-b221-4701-a7b2-6552f08320da\"}],\"packageUris\":[\"http://schema.mathworks.com/mf0/Connector/R2020b\"],\"version\":\"1.0\"}"
  suma2_3 : My_FI_Operations/suma2_  SystemSampleTime=-1  VariantActivationTime=update diagram  Latency=0  AutoFrameSizeCalculation=off
      settings: PortSchema="{\"entries\":[{\"content\":{\"sides\":[{\"content\":{\"connectorIds\":[\"Out1\"]},\"type\":\"ConnectorPlacement.EquallySpacedRectSide\",\"uuid\":\"423828e0-6700-4575-ac06-a5fb7cb5569f\"},{\"content\":{\"connectorIds\":[\"In2\"],\"side\":\"RIGHT\"},\"type\":\"ConnectorPlacement.EquallySpacedRectSide\",\"uuid\":\"a42db842-eb55-44f2-8f04-0144bc45d908\"},{\"content\":{\"connectorIds\":[\"In1\"],\"side\":\"TOP\"},\"type\":\"ConnectorPlacement.EquallySpacedRectSide\",\"uuid\":\"eef5137d-31f0-46b4-a53b-5aa31464a7f9\"}]},\"type\":\"ConnectorPlacement.EquallySpacedConnector\",\"uuid\":\"7dd7fe03-b221-4701-a7b2-6552f08320da\"}],\"packageUris\":[\"http://schema.mathworks.com/mf0/Connector/R2020b\"],\"version\":\"1.0\"}"
  suma4_3 : My_FI_Operations/suma4_  SystemSampleTime=-1  VariantActivationTime=update diagram  Latency=0  AutoFrameSizeCalculation=off
      settings: PortSchema="{\"entries\":[{\"content\":{\"sides\":[{\"content\":{\"connectorIds\":[\"Out1\"]},\"type\":\"ConnectorPlacement.EquallySpacedRectSide\",\"uuid\":\"423828e0-6700-4575-ac06-a5fb7cb5569f\"},{\"content\":{\"connectorIds\":[\"In2\"],\"side\":\"RIGHT\"},\"type\":\"ConnectorPlacement.EquallySpacedRectSide\",\"uuid\":\"a42db842-eb55-44f2-8f04-0144bc45d908\"},{\"content\":{\"connectorIds\":[\"In1\"],\"side\":\"TOP\"},\"type\":\"ConnectorPlacement.EquallySpacedRectSide\",\"uuid\":\"eef5137d-31f0-46b4-a53b-5aa31464a7f9\"}]},\"type\":\"ConnectorPlacement.EquallySpacedConnector\",\"uuid\":\"7dd7fe03-b221-4701-a7b2-6552f08320da\"}],\"packageUris\":[\"http://schema.mathworks.com/mf0/Connector/R2020b\"],\"version\":\"1.0\"}"
  suma6_3 : My_FI_Operations/suma6_  SystemSampleTime=-1  VariantActivationTime=update diagram  Latency=0  AutoFrameSizeCalculation=off
      settings: PortSchema="{\"entries\":[{\"content\":{\"sides\":[{\"content\":{\"connectorIds\":[\"Out1\"]},\"type\":\"ConnectorPlacement.EquallySpacedRectSide\",\"uuid\":\"423828e0-6700-4575-ac06-a5fb7cb5569f\"},{\"content\":{\"connectorIds\":[\"In2\"],\"side\":\"RIGHT\"},\"type\":\"ConnectorPlacement.EquallySpacedRectSide\",\"uuid\":\"a42db842-eb55-44f2-8f04-0144bc45d908\"},{\"content\":{\"connectorIds\":[\"In1\"],\"side\":\"TOP\"},\"type\":\"ConnectorPlacement.EquallySpacedRectSide\",\"uuid\":\"eef5137d-31f0-46b4-a53b-5aa31464a7f9\"}]},\"type\":\"ConnectorPlacement.EquallySpacedConnector\",\"uuid\":\"7dd7fe03-b221-4701-a7b2-6552f08320da\"}],\"packageUris\":[\"http://schema.mathworks.com/mf0/Connector/R2020b\"],\"version\":\"1.0\"}"
  sumd-2_3 : My_FI_Operations/sumd-2_  SystemSampleTime=-1  VariantActivationTime=update diagram  Latency=0  AutoFrameSizeCalculation=off
      settings: PortSchema="{\"entries\":[{\"content\":{\"sides\":[{\"content\":{\"connectorIds\":[]},\"type\":\"ConnectorPlacement.EquallySpacedRectSide\",\"uuid\":\"423828e0-6700-4575-ac06-a5fb7cb5569f\"},{\"content\":{\"connectorIds\":[\"In2\"],\"side\":\"RIGHT\"},\"type\":\"ConnectorPlacement.EquallySpacedRectSide\",\"uuid\":\"a42db842-eb55-44f2-8f04-0144bc45d908\"},{\"content\":{\"connectorIds\":[\"Out1\"],\"side\":\"TOP\"},\"type\":\"ConnectorPlacement.EquallySpacedRectSide\",\"uuid\":\"eef5137d-31f0-46b4-a53b-5aa31464a7f9\"},{\"content\":{\"connectorIds\":[\"In1\"],\"side\":\"BOTTOM\"},\"type\":\"ConnectorPlacement.EquallySpacedRectSide\",\"uuid\":\"0a29e77a-4bdf-45d0-8a25-1103c3446174\"}]},\"type\":\"ConnectorPlacement.EquallySpacedConnector\",\"uuid\":\"7dd7fe03-b221-4701-a7b2-6552f08320da\"}],\"packageUris\":[\"http://schema.mathworks.com/mf0/Connector/R2020b\"],\"version\":\"1.0\"}"
  sumin_3 : My_FI_Operations/sumin_  SystemSampleTime=-1  VariantActivationTime=update diagram  Latency=0  AutoFrameSizeCalculation=off
      settings: PortSchema="{\"entries\":[{\"content\":{\"sides\":[{\"content\":{\"connectorIds\":[\"In1\"]},\"type\":\"ConnectorPlacement.EquallySpacedRectSide\",\"uuid\":\"423828e0-6700-4575-ac06-a5fb7cb5569f\"},{\"content\":{\"connectorIds\":[\"Out1\"],\"side\":\"RIGHT\"},\"type\":\"ConnectorPlacement.EquallySpacedRectSide\",\"uuid\":\"a42db842-eb55-44f2-8f04-0144bc45d908\"},{\"content\":{\"connectorIds\":[],\"side\":\"TOP\"},\"type\":\"ConnectorPlacement.EquallySpacedRectSide\",\"uuid\":\"eef5137d-31f0-46b4-a53b-5aa31464a7f9\"},{\"content\":{\"connectorIds\":[\"In2\"],\"side\":\"BOTTOM\"},\"type\":\"ConnectorPlacement.EquallySpacedRectSide\",\"uuid\":\"f3760898-0e2b-4385-8757-2cc61988fa54\"}]},\"type\":\"ConnectorPlacement.EquallySpacedConnector\",\"uuid\":\"7dd7fe03-b221-4701-a7b2-6552f08320da\"}],\"packageUris\":[\"http://schema.mathworks.com/mf0/Connector/R2020b\"],\"version\":\"1.0\"}"
  sumq-1_3 : My_FI_Operations/sumq-1_  SystemSampleTime=-1  VariantActivationTime=update diagram  Latency=0  AutoFrameSizeCalculation=off
      settings: PortSchema="{\"entries\":[{\"content\":{\"sides\":[{\"content\":{\"connectorIds\":[]},\"type\":\"ConnectorPlacement.EquallySpacedRectSide\",\"uuid\":\"423828e0-6700-4575-ac06-a5fb7cb5569f\"},{\"content\":{\"connectorIds\":[\"In2\"],\"side\":\"RIGHT\"},\"type\":\"ConnectorPlacement.EquallySpacedRectSide\",\"uuid\":\"a42db842-eb55-44f2-8f04-0144bc45d908\"},{\"content\":{\"connectorIds\":[\"Out1\"],\"side\":\"TOP\"},\"type\":\"ConnectorPlacement.EquallySpacedRectSide\",\"uuid\":\"eef5137d-31f0-46b4-a53b-5aa31464a7f9\"},{\"content\":{\"connectorIds\":[\"In1\"],\"side\":\"BOTTOM\"},\"type\":\"ConnectorPlacement.EquallySpacedRectSide\",\"uuid\":\"2873f229-5340-47da-9b40-109923f96826\"}]},\"type\":\"ConnectorPlacement.EquallySpacedConnector\",\"uuid\":\"7dd7fe03-b221-4701-a7b2-6552f08320da\"}],\"packageUris\":[\"http://schema.mathworks.com/mf0/Connector/R2020b\"],\"version\":\"1.0\"}"
  Out1 : Outport
  Out2 : Outport  Port=2
  Out3 : Outport  Port=3
  wires:
  multa8_3/1 -> Delay88/1
  multa6_3/1 -> suma6_3/1
  Delay84/1 -> suma2_3/2
  sumin_3/1 -> multa2_3/2, multa4_3/2, multa6_3/2, multa8_3/2, multa10_3/2, multa12_3/2, Zero-Order Hold8/1
  multa12_3/1 -> Delay80/1
  In3/1 -> sumd-2_3/1
  suma6_3/1 -> Delay85/1
  Delay85/1 -> Delay81/1
  sumd-2_3/1 -> sumq-1_3/1
  a4_3/1 -> multa4_3/1
  sumq-1_3/1 -> sumin_3/2
  a10_3/1 -> multa10_3/1
  Zero-Order Hold8/1 -> Out1/1
  Delay88/1 -> Delay84/1
  Delay89/1 -> suma6_3/2
  multa2_3/1 -> suma2_3/1
  a12_3/1 -> multa12_3/1
  multa10_3/1 -> Delay90/1
  Delay87/1 -> suma4_3/2
  Delay90/1 -> Delay87/1
  Delay80/1 -> Delay89/1
  a6_3/1 -> multa6_3/1
  a8_3/1 -> multa8_3/1
  a2_3/1 -> multa2_3/1
  multa4_3/1 -> suma4_3/1
  suma2_3/1 -> Out3/1
  In2/1 -> sumq-1_3/2
  suma4_3/1 -> Out2/1
  In1/1 -> Delay109/1
  Delay109/1 -> sumin_3/1
  Delay81/1 -> sumd-2_3/2

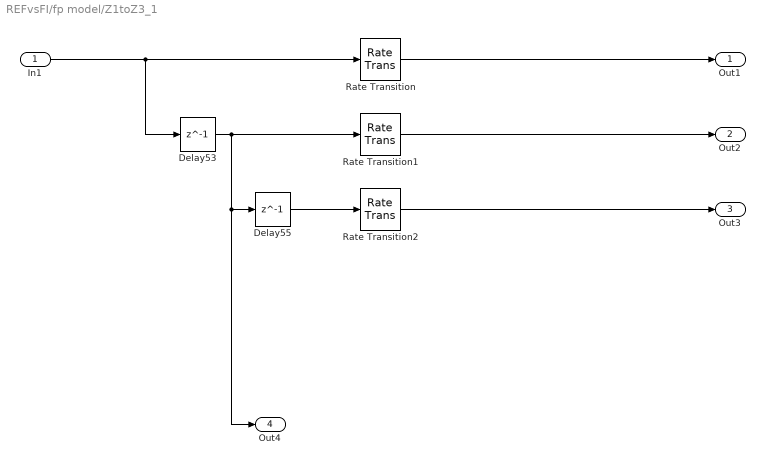
== system REFvsFI/fp model/Z1toZ3_1 ==
  In1 : Inport
  Delay53 : Delay  DelayLength=1  SampleTime=Ts
  Delay55 : Delay  DelayLength=1  SampleTime=Ts
  Rate Transition : RateTransition  OutPortSampleTime=3*Ts
  Rate Transition1 : RateTransition  OutPortSampleTime=3*Ts
  Rate Transition2 : RateTransition  OutPortSampleTime=3*Ts
  Out1 : Outport
  Out2 : Outport  Port=2
  Out3 : Outport  Port=3
  Out4 : Outport  Port=4
  wires:
  Delay53/1 -> Rate Transition1/1, Out4/1, Delay55/1
  Delay55/1 -> Rate Transition2/1
  In1/1 -> Delay53/1, Rate Transition/1
  Rate Transition/1 -> Out1/1
  Rate Transition1/1 -> Out2/1
  Rate Transition2/1 -> Out3/1

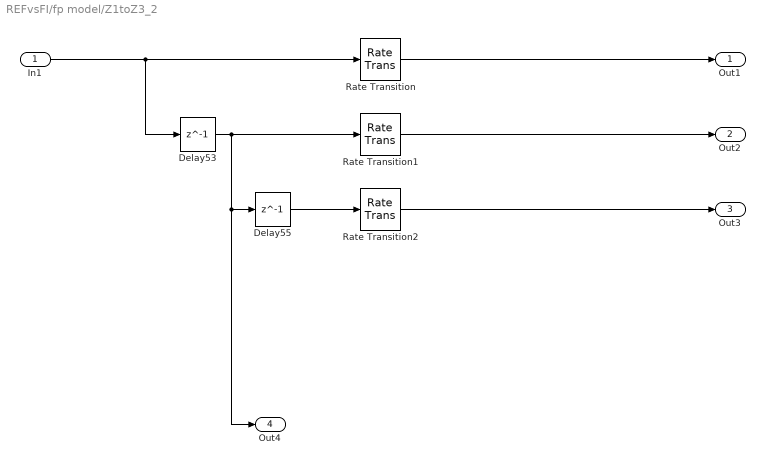
== system REFvsFI/fp model/Z1toZ3_2 ==
  In1 : Inport
  Delay53 : Delay  DelayLength=1  SampleTime=Ts
  Delay55 : Delay  DelayLength=1  SampleTime=Ts
  Rate Transition : RateTransition  OutPortSampleTime=3*Ts
  Rate Transition1 : RateTransition  OutPortSampleTime=3*Ts
  Rate Transition2 : RateTransition  OutPortSampleTime=3*Ts
  Out1 : Outport
  Out2 : Outport  Port=2
  Out3 : Outport  Port=3
  Out4 : Outport  Port=4
  wires:
  Delay53/1 -> Rate Transition1/1, Out4/1, Delay55/1
  Delay55/1 -> Rate Transition2/1
  In1/1 -> Delay53/1, Rate Transition/1
  Rate Transition/1 -> Out1/1
  Rate Transition1/1 -> Out2/1
  Rate Transition2/1 -> Out3/1

== system REFvsFI/fp model/Z1toZ3_3 ==
  In1 : Inport
  Delay53 : Delay  DelayLength=1  SampleTime=Ts
  Delay55 : Delay  DelayLength=1  SampleTime=Ts
  Rate Transition : RateTransition  OutPortSampleTime=3*Ts
  Rate Transition1 : RateTransition  OutPortSampleTime=3*Ts
  Rate Transition2 : RateTransition  OutPortSampleTime=3*Ts
  Out1 : Outport
  Out2 : Outport  Port=2
  Out3 : Outport  Port=3
  Out4 : Outport  Port=4
  wires:
  Delay53/1 -> Rate Transition1/1, Out4/1, Delay55/1
  Delay55/1 -> Rate Transition2/1
  In1/1 -> Delay53/1, Rate Transition/1
  Rate Transition/1 -> Out1/1
  Rate Transition1/1 -> Out2/1
  Rate Transition2/1 -> Out3/1

== system REFvsFI/ref model/multa10_1 ==
  In2 : Inport
  In1 : Inport  Port=2
  Product : Product  OutDataTypeStr=double  RndMeth=Nearest
  Out1 : Outport
  wires:
  Product/1 -> Out1/1
  In2/1 -> Product/2
  In1/1 -> Product/1

== system REFvsFI/ref model/multa10_2 ==
  In2 : Inport
  In1 : Inport  Port=2
  Product : Product  OutDataTypeStr=double  RndMeth=Nearest
  Out1 : Outport
  wires:
  Product/1 -> Out1/1
  In2/1 -> Product/2
  In1/1 -> Product/1

== system REFvsFI/ref model/multa10_3 ==
  In2 : Inport
  In1 : Inport  Port=2
  Product : Product  OutDataTypeStr=double  RndMeth=Nearest
  Out1 : Outport
  wires:
  Product/1 -> Out1/1
  In2/1 -> Product/2
  In1/1 -> Product/1

== system REFvsFI/ref model/multa12_1 ==
  In2 : Inport
  In1 : Inport  Port=2
  Product : Product  OutDataTypeStr=double  RndMeth=Nearest
  Out1 : Outport
  wires:
  Product/1 -> Out1/1
  In1/1 -> Product/1
  In2/1 -> Product/2

== system REFvsFI/ref model/multa12_2 ==
  In2 : Inport
  In1 : Inport  Port=2
  Product : Product  OutDataTypeStr=double  RndMeth=Nearest
  Out1 : Outport
  wires:
  Product/1 -> Out1/1
  In1/1 -> Product/1
  In2/1 -> Product/2

== system REFvsFI/ref model/multa12_3 ==
  In2 : Inport
  In1 : Inport  Port=2
  Product : Product  OutDataTypeStr=double  RndMeth=Nearest
  Out1 : Outport
  wires:
  Product/1 -> Out1/1
  In1/1 -> Product/1
  In2/1 -> Product/2

== system REFvsFI/ref model/multa2_1 ==
  In2 : Inport
  In1 : Inport  Port=2
  Product : Product  OutDataTypeStr=double  RndMeth=Nearest
  Out1 : Outport
  wires:
  Product/1 -> Out1/1
  In1/1 -> Product/1
  In2/1 -> Product/2

== system REFvsFI/ref model/multa2_2 ==
  In2 : Inport
  In1 : Inport  Port=2
  Product : Product  OutDataTypeStr=double  RndMeth=Nearest
  Out1 : Outport
  wires:
  Product/1 -> Out1/1
  In1/1 -> Product/1
  In2/1 -> Product/2

== system REFvsFI/ref model/multa2_3 ==
  In2 : Inport
  In1 : Inport  Port=2
  Product : Product  OutDataTypeStr=double  RndMeth=Nearest
  Out1 : Outport
  wires:
  Product/1 -> Out1/1
  In1/1 -> Product/1
  In2/1 -> Product/2

== system REFvsFI/ref model/multa4_1 ==
  In2 : Inport
  In1 : Inport  Port=2
  Product : Product  OutDataTypeStr=double  RndMeth=Nearest
  Out1 : Outport
  wires:
  In2/1 -> Product/2
  Product/1 -> Out1/1
  In1/1 -> Product/1

== system REFvsFI/ref model/multa4_2 ==
  In2 : Inport
  In1 : Inport  Port=2
  Product : Product  OutDataTypeStr=double  RndMeth=Nearest
  Out1 : Outport
  wires:
  In2/1 -> Product/2
  Product/1 -> Out1/1
  In1/1 -> Product/1

== system REFvsFI/ref model/multa4_3 ==
  In2 : Inport
  In1 : Inport  Port=2
  Product : Product  OutDataTypeStr=double  RndMeth=Nearest
  Out1 : Outport
  wires:
  In2/1 -> Product/2
  Product/1 -> Out1/1
  In1/1 -> Product/1

== system REFvsFI/ref model/multa6_1 ==
  In2 : Inport
  In1 : Inport  Port=2
  Product : Product  OutDataTypeStr=double  RndMeth=Nearest
  Out1 : Outport
  wires:
  Product/1 -> Out1/1
  In2/1 -> Product/2
  In1/1 -> Product/1

== system REFvsFI/ref model/multa6_2 ==
  In2 : Inport
  In1 : Inport  Port=2
  Product : Product  OutDataTypeStr=double  RndMeth=Nearest
  Out1 : Outport
  wires:
  Product/1 -> Out1/1
  In2/1 -> Product/2
  In1/1 -> Product/1

== system REFvsFI/ref model/multa6_3 ==
  In2 : Inport
  In1 : Inport  Port=2
  Product : Product  OutDataTypeStr=double  RndMeth=Nearest
  Out1 : Outport
  wires:
  Product/1 -> Out1/1
  In2/1 -> Product/2
  In1/1 -> Product/1

== system REFvsFI/ref model/multa8_1 ==
  In2 : Inport
  In1 : Inport  Port=2
  Product : Product  OutDataTypeStr=double  RndMeth=Nearest
  Out1 : Outport
  wires:
  Product/1 -> Out1/1
  In2/1 -> Product/2
  In1/1 -> Product/1

== system REFvsFI/ref model/multa8_2 ==
  In2 : Inport
  In1 : Inport  Port=2
  Product : Product  OutDataTypeStr=double  RndMeth=Nearest
  Out1 : Outport
  wires:
  Product/1 -> Out1/1
  In2/1 -> Product/2
  In1/1 -> Product/1

== system REFvsFI/ref model/multa8_3 ==
  In2 : Inport
  In1 : Inport  Port=2
  Product : Product  OutDataTypeStr=double  RndMeth=Nearest
  Out1 : Outport
  wires:
  Product/1 -> Out1/1
  In2/1 -> Product/2
  In1/1 -> Product/1
